simulink model "AFEFV_RC_2L"  (R2013a)
settings: Solver=FixedStepDiscrete  SolverMode=SingleTasking  StartTime=0.0  StopTime=5  FixedStep=Tpas  RelTol=1e-3
InitFcn:
  |  AFE_2L_RC_param_DT1
values from neighbouring files (symbols this model uses):
  Freq = 50    [AFE_2L_RC_param_DT1.m]    (also in AFE_FV_Params.m; AFE_PontHPV2.m; AFEsimplepara.m; AFEsimpleparaDT1.m)
  hys = 100    [AFE_2L_RC_param_DT1.m]    (also in AFE_FV_Params.m = 150; AFE_PontHPV2.m = 150; AFEsimplepara.m = 0.1; AFEsimpleparaDT1.m)
  I = (P+Numd(2)/Dend(1))/Ts    [AFE_2L_RC_param_DT1.m]    (also in AFE_PontHPV2.m; AFEsimpleparaDT1.m; AFEsimpleparaPV2.m; initAFE_PontHPV3.m)
  Imax = 1300    [AFE_2L_RC_param_DT1.m]    (also in AFE_FV_Params.m = 1500; AFEsimpleparaDT1.m = 5000; AFEsimpleparaPV2.m = 5000)
  P = Numd(1)/Dend(1)    [AFE_2L_RC_param_DT1.m]    (also in AFE_PontHPV2.m; AFEsimpleparaDT1.m; AFEsimpleparaPV2.m; initAFE_PontHPV3.m)
  Rac = 2.5    [AFEsimplepara.m]
  Tpas = 5e-5    (= 5e-05)    [AFE_2L_RC_param_DT1.m]    (also in AFE_FV_Params.m; AFE_PontHPV2.m = 3e-06; AFEsimplepara.m = 1e-05; AFEsimpleparaDT1.m)
  Vac = 2000    [AFE_2L_RC_param_DT1.m]    (also in AFE_FV_Params.m; AFE_PontHPV2.m; AFEsimplepara.m; AFEsimpleparaDT1.m)
libraries: powerlib x22, simulink x8, powerlib_meascontrol x2
settings Model: Creator=LiberT  LastModifiedBy=Francis
settings DataIOCC: SignalLoggingSaveFormat=ModelDataLogs
settings OptimizationCC: ExpressionDepthLimit=2147483647
settings DebuggingCC: MultiTaskDSMMsg=warning  MultiTaskCondExecSysMsg=none  FcnCallInpInsideContextMsg=EnableAllAsWarning  StrictBusMsg=None
settings RTWCC: IncludeERTFirstTime=on

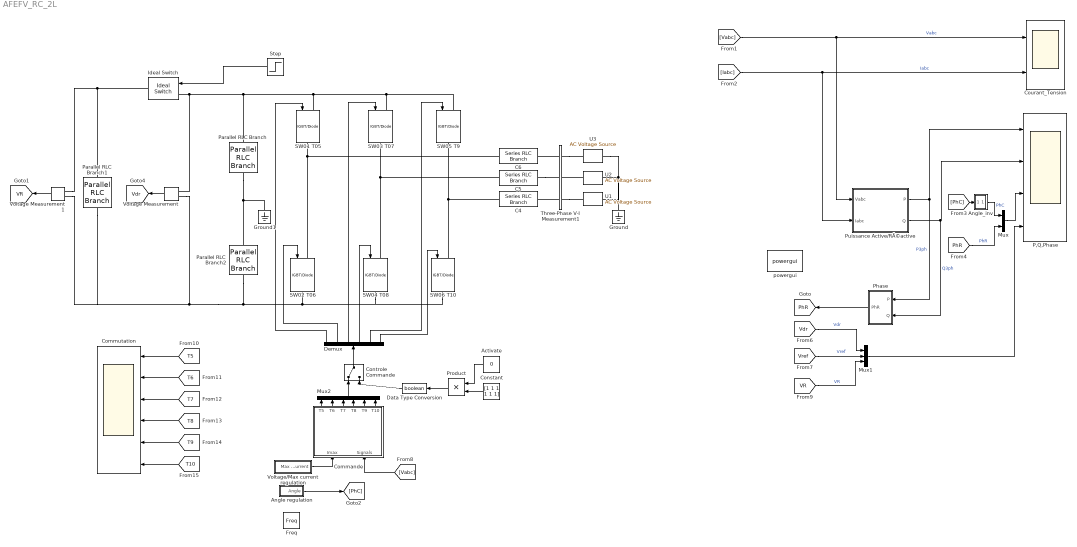
== system AFEFV_RC_2L ==
  Activate : Constant  Value=0
  Angle regulation : Subsystem
  Angle_inv : Subsystem
  C4 : powerlib/Elements/Series RLC Branch  LConnTagsString=__new0  RConnTagsString=__new0  BranchType=L  Resistance=Rac  Inductance=3e-3  SetiL0=off  InitialCurrent=0  Capacitance=300e-3  Setx0=off  InitialVoltage=0  Measurements=None
  C5 : powerlib/Elements/Series RLC Branch  LConnTagsString=__new0  RConnTagsString=__new0  BranchType=L  Resistance=Rac  Inductance=3e-3  SetiL0=off  InitialCurrent=0  Capacitance=300e-3  Setx0=off  InitialVoltage=0  Measurements=None
  C6 : powerlib/Elements/Series RLC Branch  LConnTagsString=__new0  RConnTagsString=__new0  BranchType=L  Resistance=Rac  Inductance=3e-3  SetiL0=off  InitialCurrent=0  Capacitance=300e-3  Setx0=off  InitialVoltage=0  Measurements=None
  Commande : Subsystem
  Commutation : Scope  NumInputPorts=6
      settings: TickLabels=on  TimeRange=3.615  YMin=-0.2~-0.2~-0.2~-0.2~-0.2~-0.2  YMax=1.2~1.2~1.2~1.2~1.2~1.2  SaveName=PQ_Phi1  MaxDataPoints=50000
  Constant : Constant  Value=[1 1 1 1 1 1]
  Controle Commande : ManualSwitch
  Courant_Tension : Scope  NumInputPorts=2
      settings: TickLabels=on  TimeRange=0.04  YMin=-1750~-1500  YMax=1750~1500  SaveName=Courant_Tension
  Data Type Conversion : DataTypeConversion  OutDataTypeStr=boolean
  Demux : Demux  Outputs=6
  Freq : Constant  Value=Freq  SampleTime=Tpas
  Ground : powerlib/Elements/Ground  LConnTagsString=a
  Ground1 : powerlib/Elements/Ground  LConnTagsString=a
  Ideal Switch : powerlib/Power Electronics/Ideal Switch  Ron=0.001  Lon=0  IC=0  Rs=1e5  Cs=inf  Measurements=off
  Mux : Mux  Inputs=2
  Mux1 : Mux  Inputs=3
  Mux2 : Mux  Inputs=6
  P,Q,Phase : Scope  NumInputPorts=4
      settings: TickLabels=on  ShowLegends=on  TimeRange=3.615  YMin=-500000~-2e+06~-200~0  YMax=3.5e+06~5e+06~200~5500  SaveName=PQ_Phi  MaxDataPoints=50000
  Parallel RLC Branch : powerlib/Elements/Parallel RLC Branch  LConnTagsString=a  RConnTagsString=__new0  BranchType=C  Resistance=9.26  Inductance=1e-3  SetiL0=off  InitialCurrent=0  Capacitance=330e-3*2  Setx0=on  InitialVoltage=2500  Measurements=Branch voltage
  Parallel RLC Branch1 : powerlib/Elements/Parallel RLC Branch  LConnTagsString=a  RConnTagsString=__new0  BranchType=R  Resistance=9.26  Inductance=1e-3  SetiL0=off  InitialCurrent=0  Capacitance=330e-3  Setx0=off  InitialVoltage=5000  Measurements=Branch voltage
  Parallel RLC Branch2 : powerlib/Elements/Parallel RLC Branch  LConnTagsString=a  RConnTagsString=__new0  BranchType=C  Resistance=9.26  Inductance=1e-3  SetiL0=off  InitialCurrent=0  Capacitance=330e-3*2  Setx0=on  InitialVoltage=2500  Measurements=Branch voltage
  Phase : Subsystem
  Product : Product
  Puissance Active/RÃ©active : Subsystem
  SW01 T05 : powerlib/Power Electronics/IGBT//Diode  Ron=1e-3  Rs=1e5  Cs=Tpas  Measurements=off
  SW02 T06 : powerlib/Power Electronics/IGBT//Diode  Ron=1e-3  Rs=1e5  Cs=Tpas  Measurements=off
  SW03 T07 : powerlib/Power Electronics/IGBT//Diode  Ron=1e-3  Rs=1e5  Cs=Tpas  Measurements=off
  SW04 T08 : powerlib/Power Electronics/IGBT//Diode  Ron=1e-3  Rs=1e5  Cs=Tpas  Measurements=off
  SW05 T9 : powerlib/Power Electronics/IGBT//Diode  Ron=1e-3  Rs=1e5  Cs=Tpas  Measurements=off
  SW06 T10 : powerlib/Power Electronics/IGBT//Diode  Ron=1e-3  Rs=1e5  Cs=Tpas  Measurements=off
  Step : Step  Time=2.125  SampleTime=Tpas
  Three-Phase V-I Measurement1 : powerlib/Measurements/Three-Phase V-I Measurement  VoltageMeasurement=phase-to-ground  SetLabelV=on  LabelV=Vabc  Vpu=off  VpuLL=off  CurrentMeasurement=yes  SetLabelI=on  LabelI=Iabc  Ipu=off  Pbase=100e6  Vbase=500e3  OutputType=Complex  PhasorSimulation=off  PSBequivalent=0
  U1 : powerlib/Electrical Sources/AC Voltage Source  Amplitude=Vac*sqrt(2/3)  Phase=120  Frequency=Freq  SampleTime=0  Measurements=Voltage
  U2 : powerlib/Electrical Sources/AC Voltage Source  Amplitude=Vac*sqrt(2/3)  Phase=-120  Frequency=Freq  SampleTime=0  Measurements=Voltage
  U3 : powerlib/Electrical Sources/AC Voltage Source  Amplitude=Vac*sqrt(2/3)  Phase=0  Frequency=Freq  SampleTime=0  Measurements=Voltage
  Voltage Measurement : powerlib/Measurements/Voltage Measurement  PhasorSimulation=off  OutputType=Complex  PSBequivalent=0
  Voltage Measurement1 : powerlib/Measurements/Voltage Measurement  PhasorSimulation=off  OutputType=Complex  PSBequivalent=0
  Voltage/Max current regulation : Subsystem
  powergui : powerlib/powergui  Priority=1  SimulationMode=Discrete  SolverType=Tustin  SampleTime=Tpas  frequency=50  SPID=off  DisableSnubberDevices=off  DisableRonSwitches=off  DisableVfSwitches=off  SwTol=0  Interpol=off  DisplayEquations=off  frequencyindice=50  Pbase=100e6  ErrMax=1e-4  Iterations=50  UnitsV=kV  UnitsW=MW  FunctionMessages=off  echomessages=off  HookPort=off  EnableUseOfTLC=off  x0status=blocks  RestoreLinks=warning  ResistiveCurrentMeasurement=off  Frange=[0:2:500]  Ylog=off  Xlog=on  ShowGrid=off  save=off  variable=ZData  structure=Courant_Tension  ZoomFFT=off  StartTime=4.75005  cycles=12  DisplayStyle=2  fundamental=50  FreqAxis=off  MaxFrequency=2000  frequencyindicesteady=1  RmsSteady=1  display=off  Ts=0  methode=off
  tag scope: PhR=global, VR=global, Vdr=global
  wires:
  [Iabc] -> Puissance Active/RÃ©active/2(Iabc), Courant_Tension/2  "Iabc"
  [Vabc] -> Puissance Active/RÃ©active/1(Vabc), Courant_Tension/1  "Vabc"
  Puissance Active/RÃ©active/1(P) -> P,Q,Phase/1, Phase/1(P)  "P3ph"
  Phase/1(PhR) -> [PhR]
  [PhC] -> Angle_inv/1(Angle_in)
  [PhR] -> Mux/2  "PhR"
  Mux/1 -> P,Q,Phase/3
  Puissance Active/RÃ©active/2(Q) -> Phase/2(Q), P,Q,Phase/2  "Q3ph"
  Angle_inv/1(Angle_out) -> Mux/1  "PhC"
  Voltage Measurement/1 -> [Vdr]
  [Vdr] -> Mux1/1  "Vdr"
  [Vref] -> Mux1/2  "Vref"
  Mux1/1 -> P,Q,Phase/4
  [VR] -> Mux1/3  "VR"
  Angle regulation/1(Angle) -> [PhC]
  Voltage Measurement1/1 -> [VR]
  [Vabc] -> Commande/2("Signals ")
  Voltage/Max current regulation/1(Max Current) -> Commande/1(Imax)
  Demux/1 -> SW01 T05/1
  Demux/2 -> SW02 T06/1
  Demux/3 -> SW03 T07/1
  Demux/4 -> SW04 T08/1
  Demux/5 -> SW05 T9/1
  Demux/6 -> SW06 T10/1
  Commande/1(T5) -> Mux2/1
  Commande/2(T6) -> Mux2/2
  Commande/3(T7) -> Mux2/3
  Commande/4(T8) -> Mux2/4
  Commande/5(T9) -> Mux2/5
  Commande/6(T10) -> Mux2/6
  Controle Commande/1 -> Demux/1
  Mux2/1 -> Controle Commande/1
  Data Type Conversion/1 -> Controle Commande/2
  [T5] -> Commutation/1
  [T6] -> Commutation/2
  [T7] -> Commutation/3
  [T8] -> Commutation/4
  [T9] -> Commutation/5
  [T10] -> Commutation/6
  Constant/1 -> Product/2
  Product/1 -> Data Type Conversion/1
  Activate/1 -> Product/1
  Step/1 -> Ideal Switch/1
  connections:
  Voltage Measurement/LConn2 -- Parallel RLC Branch2/RConn1 -- SW02 T06/RConn1 -- SW06 T10/RConn1 -- SW04 T08/RConn1 -- Parallel RLC Branch1/RConn1 -- Voltage Measurement1/LConn2
  SW02 T06/LConn1 -- C6/LConn1 -- SW01 T05/RConn1
  SW06 T10/LConn1 -- SW05 T9/RConn1 -- C4/LConn1
  SW04 T08/LConn1 -- C5/LConn1 -- SW03 T07/RConn1
  U2/LConn1 -- U1/LConn1 -- Ground/LConn1 -- U3/LConn1
  SW01 T05/LConn1 -- Parallel RLC Branch/LConn1 -- Voltage Measurement/LConn1 -- Ideal Switch/LConn1 -- SW05 T9/LConn1 -- SW03 T07/LConn1
  Parallel RLC Branch2/LConn1 -- Parallel RLC Branch/RConn1 -- Ground1/LConn1
  Voltage Measurement1/LConn1 -- Ideal Switch/RConn1 -- Parallel RLC Branch1/LConn1
  Three-Phase V-I Measurement1/LConn1 -- C6/RConn1
  Three-Phase V-I Measurement1/RConn1 -- U3/RConn1
  U2/RConn1 -- Three-Phase V-I Measurement1/RConn2
  C5/RConn1 -- Three-Phase V-I Measurement1/LConn2
  Three-Phase V-I Measurement1/LConn3 -- C4/RConn1
  Three-Phase V-I Measurement1/RConn3 -- U1/RConn1

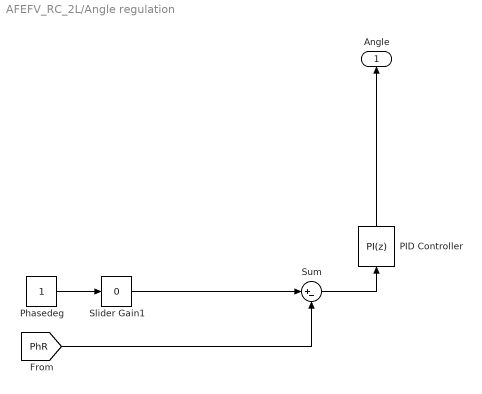
== system AFEFV_RC_2L/Angle regulation ==
  PID Controller : simulink/Continuous/PID Controller  Controller=PI  TimeDomain=Discrete-time  SampleTime=Tpas  IntegratorMethod=Forward Euler  FilterMethod=Forward Euler  Form=Parallel  P=P  I=I  D=0  N=100  InitialConditionSource=internal  InitialConditionForIntegrator=0  InitialConditionForFilter=0  ExternalReset=none  LimitOutput=off  UpperSaturationLimit=179.5  LowerSaturationLimit=-179.5  LinearizeAsGain=on  AntiWindupMode=clamping  Kb=1  TrackingMode=off  Kt=1  PParamMin=[]  PParamMax=[]  IParamMin=[]  IParamMax=[]  DParamMin=[]  DParamMax=[]  NParamMin=[]  NParamMax=[]  KbParamMin=[]  KbParamMax=[]  KtParamMin=[]  KtParamMax=[]  POutMin=[]  POutMax=[]  IOutMin=[]  IOutMax=[]  DOutMin=[]  DOutMax=[]  NOutMin=[]  NOutMax=[]  KbOutMin=[]  KbOutMax=[]  KtOutMin=[]  KtOutMax=[]  IntegratorOutMin=[]  IntegratorOutMax=[]  FilterOutMin=[]  FilterOutMax=[]  SumOutMin=[]  SumOutMax=[]  SumI1OutMin=[]  SumI1OutMax=[]  SumI2OutMin=[]  SumI2OutMax=[]  SumI3OutMin=[]  SumI3OutMax=[]  SumDOutMin=[]  SumDOutMax=[]  SaturationOutMin=[]  SaturationOutMax=[]  IntegratorContinuousStateAttributes=''  IntegratorStateMustResolveToSignalObject=off  IntegratorRTWStateStorageClass=Auto  FilterContinuousStateAttributes=''  FilterStateMustResolveToSignalObject=off  FilterRTWStateStorageClass=Auto
  Phasedeg : Constant  SampleTime=Tpas
  Slider Gain1 : simulink/Math Operations/Slider Gain  low=-180  gain=0  high=180
  Sum : Sum  Inputs=|+-
  Angle : Outport
  wires:
  PID Controller/1 -> Angle/1
  Slider Gain1/1 -> Sum/1
  Sum/1 -> PID Controller/1
  [PhR] -> Sum/2
  Phasedeg/1 -> Slider Gain1/1

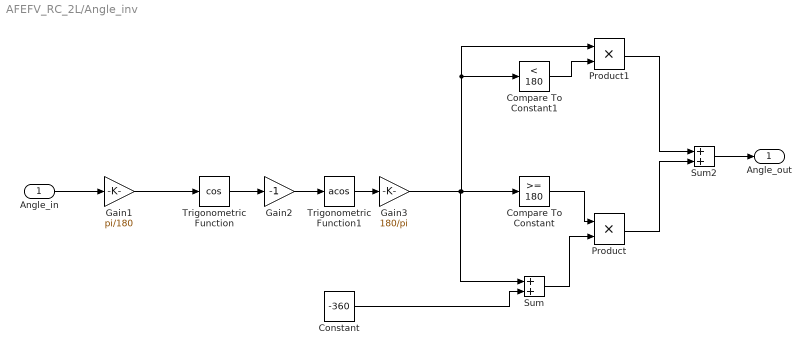
== system AFEFV_RC_2L/Angle_inv ==
  Angle_in : Inport
  Compare To Constant : simulink/Logic and Bit Operations/Compare To Constant  relop=>=  const=180  OutDataTypeStr=boolean
  Compare To Constant1 : simulink/Logic and Bit Operations/Compare To Constant  relop=<  const=180  OutDataTypeStr=boolean
  Constant : Constant  Value=-360  SampleTime=Tpas
  Gain1 : Gain  Gain=pi/180
  Gain2 : Gain  Gain=-1
  Gain3 : Gain  Gain=180/pi
  Product : Product
  Product1 : Product
  Sum : Sum
  Sum2 : Sum
  Trigonometric Function : Trigonometry  Operator=cos
  Trigonometric Function1 : Trigonometry  Operator=acos
  Angle_out : Outport
  wires:
  Compare To Constant/1 -> Product/1
  Compare To Constant1/1 -> Product1/2
  Constant/1 -> Sum/2
  Sum/1 -> Product/2
  Product/1 -> Sum2/2
  Product1/1 -> Sum2/1
  Gain1/1 -> Trigonometric Function/1
  Trigonometric Function/1 -> Gain2/1
  Gain2/1 -> Trigonometric Function1/1
  Trigonometric Function1/1 -> Gain3/1
  Sum2/1 -> Angle_out/1
  Angle_in/1 -> Gain1/1
  Gain3/1 -> Sum/1, Product1/1, Compare To Constant1/1, Compare To Constant/1

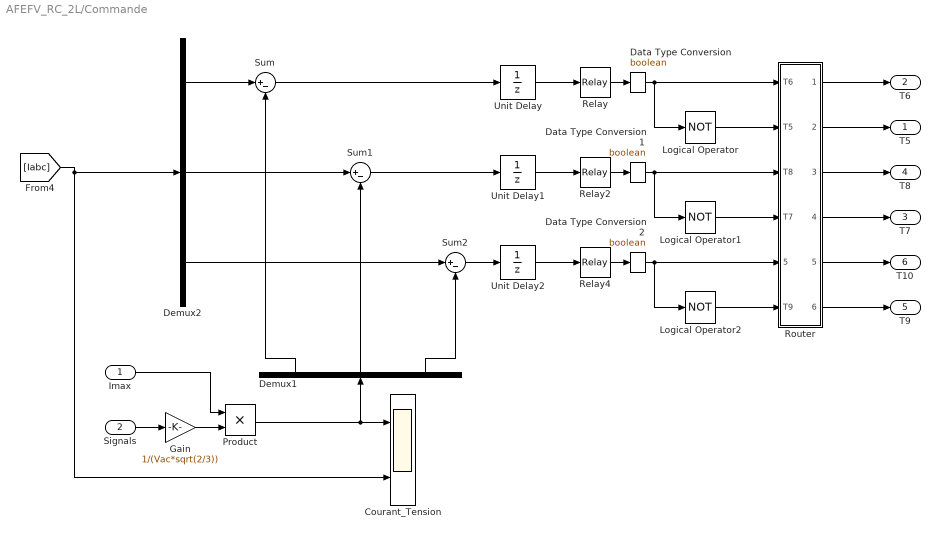
== system AFEFV_RC_2L/Commande ==
  Imax : Inport
  "Signals " : Inport  Port=2
  Courant_Tension : Scope  NumInputPorts=2
      settings: TickLabels=on  TimeRange=5  YMin=-1000~-1.75e+06  YMax=1000~3.25e+06  SaveName=Courant_Tension1  MaxDataPoints=500000
  Data Type Conversion : DataTypeConversion  OutDataTypeStr=boolean
  Data Type Conversion1 : DataTypeConversion  OutDataTypeStr=boolean
  Data Type Conversion2 : DataTypeConversion  OutDataTypeStr=boolean
  Demux1 : Demux  Outputs=3
  Demux2 : Demux  Outputs=3
  Gain : Gain  Gain=1/(Vac*sqrt(2/3))
  Logical Operator : Logic  Operator=NOT  AllPortsSameDT=off
  Logical Operator1 : Logic  Operator=NOT  AllPortsSameDT=off
  Logical Operator2 : Logic  Operator=NOT  AllPortsSameDT=off
  Product : Product
  Relay : Relay  OnSwitchValue=hys  OffSwitchValue=-hys
  Relay2 : Relay  OnSwitchValue=hys  OffSwitchValue=-hys
  Relay4 : Relay  OnSwitchValue=hys  OffSwitchValue=-hys
  Router : Subsystem
  Sum : Sum  Inputs=|+-
  Sum1 : Sum  Inputs=|+-
  Sum2 : Sum  Inputs=|+-
  Unit Delay : UnitDelay  SampleTime=-1
  Unit Delay1 : UnitDelay  SampleTime=-1
  Unit Delay2 : UnitDelay  SampleTime=-1
  T5 : Outport
  T6 : Outport  Port=2
  T7 : Outport  Port=3
  T8 : Outport  Port=4
  T9 : Outport  Port=5
  T10 : Outport  Port=6
  wires:
  Demux2/1 -> Sum/1
  Demux2/2 -> Sum1/1
  Demux2/3 -> Sum2/1
  Sum/1 -> Unit Delay/1
  Sum1/1 -> Unit Delay1/1
  Sum2/1 -> Unit Delay2/1
  Unit Delay/1 -> Relay/1
  Unit Delay1/1 -> Relay2/1
  Unit Delay2/1 -> Relay4/1
  Relay/1 -> Data Type Conversion/1
  Relay2/1 -> Data Type Conversion1/1
  Relay4/1 -> Data Type Conversion2/1
  [Iabc] -> Courant_Tension/2, Demux2/1
  Demux1/2 -> Sum1/2
  Demux1/3 -> Sum2/2
  Demux1/1 -> Sum/2
  "Signals "/1 -> Gain/1
  Gain/1 -> Product/2
  Imax/1 -> Product/1
  Product/1 -> Courant_Tension/1, Demux1/1
  Data Type Conversion/1 -> Router/1(T6), Logical Operator/1
  Data Type Conversion1/1 -> Router/3(T8), Logical Operator1/1
  Data Type Conversion2/1 -> Router/5(T10), Logical Operator2/1
  Logical Operator/1 -> Router/2(T5)
  Router/2(T5o) -> T5/1
  Router/1(T6o) -> T6/1
  Logical Operator1/1 -> Router/4(T7)
  Router/3(T8o) -> T8/1
  Router/4(T7o) -> T7/1
  Router/5(T10o) -> T10/1
  Router/6(T9o) -> T9/1
  Logical Operator2/1 -> Router/6(T9)

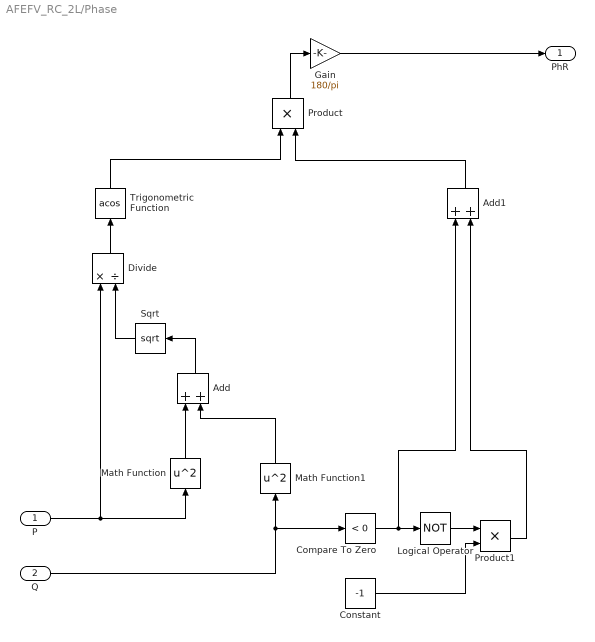
== system AFEFV_RC_2L/Phase ==
  P : Inport
  Q : Inport  Port=2
  Add : Sum
  Add1 : Sum  SampleTime=Tpas
  Compare To Zero : simulink/Logic and Bit Operations/Compare To Zero  relop=<  OutDataTypeStr=boolean
  Constant : Constant  Value=-1  SampleTime=Tpas
  Divide : Product  Inputs=*/
  Gain : Gain  Gain=180/pi  SampleTime=Tpas
  Logical Operator : Logic  Operator=NOT  AllPortsSameDT=off  OutDataTypeStr=boolean
  Math Function : Math  Operator=square  SampleTime=Tpas  SaturateOnIntegerOverflow=on
  Math Function1 : Math  Operator=square  SampleTime=Tpas  SaturateOnIntegerOverflow=on
  Product : Product
  Product1 : Product
  Sqrt : Sqrt  SaturateOnIntegerOverflow=on
  Trigonometric Function : Trigonometry  Operator=acos  SampleTime=Tpas
  PhR : Outport
  wires:
  P/1 -> Divide/1, Math Function/1
  Q/1 -> Math Function1/1, Compare To Zero/1
  Math Function/1 -> Add/1
  Math Function1/1 -> Add/2
  Add/1 -> Sqrt/1
  Sqrt/1 -> Divide/2
  Divide/1 -> Trigonometric Function/1
  Trigonometric Function/1 -> Product/1
  Compare To Zero/1 -> Add1/1, Logical Operator/1
  Logical Operator/1 -> Product1/1
  Constant/1 -> Product1/2
  Product1/1 -> Add1/2
  Add1/1 -> Product/2
  Product/1 -> Gain/1
  Gain/1 -> PhR/1

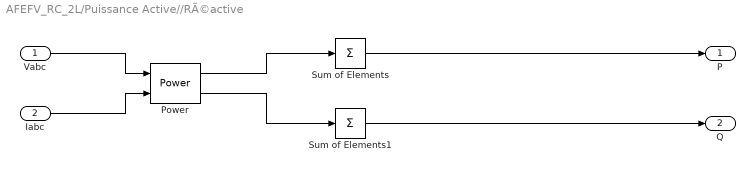
== system AFEFV_RC_2L/Puissance Active//RÃ©active ==
  Vabc : Inport
  Iabc : Inport  Port=2
  Power : powerlib_meascontrol/Measurements/Power  Freq=50  Vinit=[Vac*sqrt(2/3), 0]  Iinit=[Imax, 0]  Ts=Tpas
  Sum of Elements : Sum  Inputs=+
  Sum of Elements1 : Sum  Inputs=+
  P : Outport
  Q : Outport  Port=2
  wires:
  Power/1 -> Sum of Elements/1
  Iabc/1 -> Power/2
  Vabc/1 -> Power/1
  Power/2 -> Sum of Elements1/1
  Sum of Elements1/1 -> Q/1
  Sum of Elements/1 -> P/1

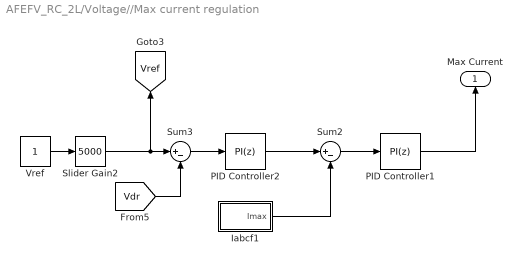
== system AFEFV_RC_2L/Voltage//Max current regulation ==
  Iabcf1 : Subsystem
  PID Controller1 : simulink/Continuous/PID Controller  Controller=PI  TimeDomain=Discrete-time  SampleTime=Tpas  IntegratorMethod=Forward Euler  FilterMethod=Forward Euler  Form=Parallel  P=5  I=0.1  D=0  N=100  InitialConditionSource=internal  InitialConditionForIntegrator=0  InitialConditionForFilter=0  ExternalReset=none  LimitOutput=on  UpperSaturationLimit=Imax  LowerSaturationLimit=0  LinearizeAsGain=on  AntiWindupMode=clamping  Kb=1  TrackingMode=off  Kt=1  PParamMin=[]  PParamMax=[]  IParamMin=[]  IParamMax=[]  DParamMin=[]  DParamMax=[]  NParamMin=[]  NParamMax=[]  KbParamMin=[]  KbParamMax=[]  KtParamMin=[]  KtParamMax=[]  POutMin=[]  POutMax=[]  IOutMin=[]  IOutMax=[]  DOutMin=[]  DOutMax=[]  NOutMin=[]  NOutMax=[]  KbOutMin=[]  KbOutMax=[]  KtOutMin=[]  KtOutMax=[]  IntegratorOutMin=[]  IntegratorOutMax=[]  FilterOutMin=[]  FilterOutMax=[]  SumOutMin=[]  SumOutMax=[]  SumI1OutMin=[]  SumI1OutMax=[]  SumI2OutMin=[]  SumI2OutMax=[]  SumI3OutMin=[]  SumI3OutMax=[]  SumDOutMin=[]  SumDOutMax=[]  SaturationOutMin=[]  SaturationOutMax=[]  IntegratorContinuousStateAttributes=''  IntegratorStateMustResolveToSignalObject=off  IntegratorRTWStateStorageClass=Auto  FilterContinuousStateAttributes=''  FilterStateMustResolveToSignalObject=off  FilterRTWStateStorageClass=Auto
  PID Controller2 : simulink/Continuous/PID Controller  Controller=PI  TimeDomain=Discrete-time  SampleTime=Tpas  IntegratorMethod=Forward Euler  FilterMethod=Forward Euler  Form=Parallel  P=5  I=20  D=0  N=100  InitialConditionSource=internal  InitialConditionForIntegrator=0  InitialConditionForFilter=0  ExternalReset=none  LimitOutput=on  UpperSaturationLimit=Imax  LowerSaturationLimit=0  LinearizeAsGain=on  AntiWindupMode=clamping  Kb=1  TrackingMode=off  Kt=1  PParamMin=[]  PParamMax=[]  IParamMin=[]  IParamMax=[]  DParamMin=[]  DParamMax=[]  NParamMin=[]  NParamMax=[]  KbParamMin=[]  KbParamMax=[]  KtParamMin=[]  KtParamMax=[]  POutMin=[]  POutMax=[]  IOutMin=[]  IOutMax=[]  DOutMin=[]  DOutMax=[]  NOutMin=[]  NOutMax=[]  KbOutMin=[]  KbOutMax=[]  KtOutMin=[]  KtOutMax=[]  IntegratorOutMin=[]  IntegratorOutMax=[]  FilterOutMin=[]  FilterOutMax=[]  SumOutMin=[]  SumOutMax=[]  SumI1OutMin=[]  SumI1OutMax=[]  SumI2OutMin=[]  SumI2OutMax=[]  SumI3OutMin=[]  SumI3OutMax=[]  SumDOutMin=[]  SumDOutMax=[]  SaturationOutMin=[]  SaturationOutMax=[]  IntegratorContinuousStateAttributes=''  IntegratorStateMustResolveToSignalObject=off  IntegratorRTWStateStorageClass=Auto  FilterContinuousStateAttributes=''  FilterStateMustResolveToSignalObject=off  FilterRTWStateStorageClass=Auto
  Slider Gain2 : simulink/Math Operations/Slider Gain  low=0  gain=5000  high=5000
  Sum2 : Sum  Inputs=|+-
  Sum3 : Sum  Inputs=|+-
  Vref : Constant  SampleTime=Tpas
  Max Current : Outport
  tag scope: Vref=global
  wires:
  Iabcf1/1(Imax) -> Sum2/2
  [Vdr] -> Sum3/2
  PID Controller1/1 -> Max Current/1
  Sum2/1 -> PID Controller1/1
  Vref/1 -> Slider Gain2/1
  Sum3/1 -> PID Controller2/1
  Slider Gain2/1 -> [Vref], Sum3/1
  PID Controller2/1 -> Sum2/1

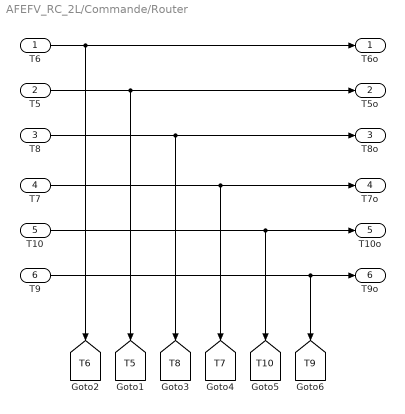
== system AFEFV_RC_2L/Commande/Router ==
  T6 : Inport
  T5 : Inport  Port=2
  T8 : Inport  Port=3
  T7 : Inport  Port=4
  T10 : Inport  Port=5
  T9 : Inport  Port=6
  T6o : Outport
  T5o : Outport  Port=2
  T8o : Outport  Port=3
  T7o : Outport  Port=4
  T10o : Outport  Port=5
  T9o : Outport  Port=6
  tag scope: T10=global, T5=global, T6=global, T7=global, T8=global, T9=global
  wires:
  T6/1 -> [T6], T6o/1
  T5/1 -> [T5], T5o/1
  T8/1 -> [T8], T8o/1
  T7/1 -> [T7], T7o/1
  T10/1 -> [T10], T10o/1
  T9/1 -> [T9], T9o/1

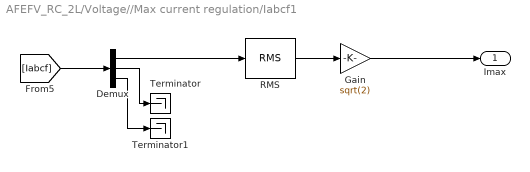
== system AFEFV_RC_2L/Voltage//Max current regulation/Iabcf1 ==
  Demux : Demux  Outputs=3
  Gain : Gain  Gain=sqrt(2)  SampleTime=Tpas
  RMS : powerlib_meascontrol/Measurements/RMS  TrueRMS=on  Freq=Freq  RMSInit=0  Ts=Tpas
  Terminator : Terminator
  Terminator1 : Terminator
  Imax : Outport
  wires:
  [Iabcf] -> Demux/1
  Demux/3 -> Terminator1/1
  Demux/2 -> Terminator/1
  Demux/1 -> RMS/1
  RMS/1 -> Gain/1
  Gain/1 -> Imax/1
